simulink model "drone"  (R2018a)
settings: Solver=ode3  StartTime=0.0  StopTime=1000  FixedStep=0.05  RelTol=1e-3  EnableMultiTasking=on
PreLoadFcn:
  | init
InitFcn:
  | init
StopFcn:
  | plots
values from neighbouring files (symbols this model uses):
  cmd_phi = 0    [init.m]
  cmd_psi = 0    [init.m]
  cmd_theta = 0    [init.m]
  cmd_z = 0    [init.m]
  deltaU1_max = Kf*4	*omega_hover_max^2    [init.m]
  deltaU1_min = Kf*4	*omega_hover_min^2    [init.m]
  deltaU2_max = Kf	*omega_hover^2    [init.m]
  deltaU3_max = Kf	*omega_hover^2    [init.m]
  deltaU4_max = Km*2	*omega_hover^2    [init.m]
  g = -9.81    [init.m]
  kd_phi = 0.5    [init.m]
  kd_psi = 0.5    [init.m]
  kd_theta = 0.5    [init.m]
  kd_z = 10    [init.m]
  Kf = 1.341e-5    (= 1.341e-05)    [init.m]
  ki_phi = 0.1    [init.m]
  ki_psi = 0.2    [init.m]
  ki_theta = 0.1    [init.m]
  ki_z = 1    [init.m]
  Km = 1.465e-6    (= 1.465e-06)    [init.m]
  kp_phi = 1    [init.m]
  kp_psi = 1    [init.m]
  kp_theta = 1    [init.m]
  kp_z = 8    [init.m]
  L = 0.235    [init.m]
  m = 1.3    [init.m]
  omega_hover_max = omega_hover + omega_hover*0.20    [init.m]
  omega_hover_min = omega_hover - omega_hover*0.10    [init.m]
undefined symbols (not defined in the file or in its folder): a, b, DiscIntNeverNeededParam
libraries: simulink x1
settings Model: Creator=Felipe Vargas  LastModifiedBy=gbs
settings DataIOCC: LimitDataPoints=on  SaveFormat=Array
settings OptimizationCC: BlockReduction=off  BufferReuse=off  LifeSpan=inf
settings DebuggingCC: AlgebraicLoopMsg=none  UnconnectedInputMsg=none  UnconnectedOutputMsg=none  UnconnectedLineMsg=none  SFUnexpectedBacktrackingDiag=warning  SFNoUnconditionalDefaultTransitionDiag=warning  SFExecutionAtInitializationDiag=none
settings HardwareCC: ProdBitPerPointer=32  ProdBitPerSizeT=32  ProdBitPerPtrDiffT=32  ProdLargestAtomicFloat=None  ProdIntDivRoundTo=Undefined  ProdEndianess=Unspecified  ProdWordSize=32  ProdHWDeviceType=32-bit Generic
settings ModelReferenceCC: PropagateSignalLabelsOutOfModel=off
settings CodeAppCC: StateflowObjectComments=on
settings GRTTargetCC: TargetLangStandard=C89/C90 (ANSI)  GeneratePreprocessorConditionals=Disable all
settings ConfigComp: CovMetricSettings=dw  CovHtmlReporting=on  CovSaveCumulativeToWorkspaceVar=on  CovSaveSingleToWorkspaceVar=on  CovExternalEMLEnable=off

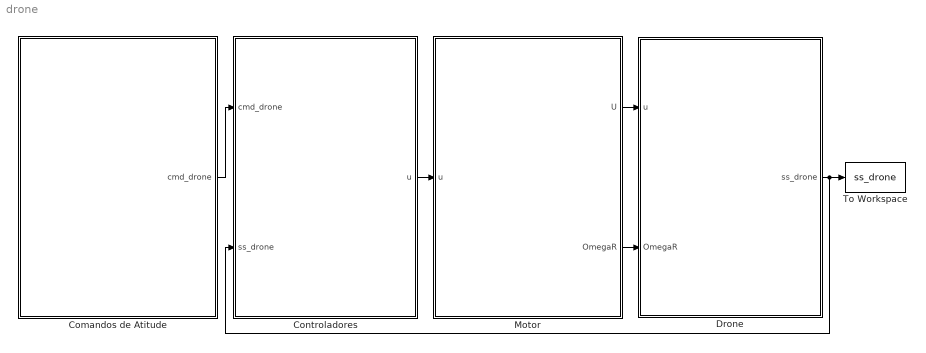
== system drone ==
  Comandos de Atitude : Subsystem
  Controladores : Subsystem
  Drone : Subsystem
  Motor : Subsystem
  To Workspace : ToWorkspace  VariableName=ss_drone  SaveFormat=Timeseries  SampleTime=-1
  wires:
  Drone/1(ss_drone) -> Controladores/2(ss_drone), To Workspace/1
  Comandos de Atitude/1(cmd_drone) -> Controladores/1(cmd_drone)
  Controladores/1(u) -> Motor/1(u)
  Motor/1(U) -> Drone/1(u)
  Motor/2(OmegaR) -> Drone/2(OmegaR)

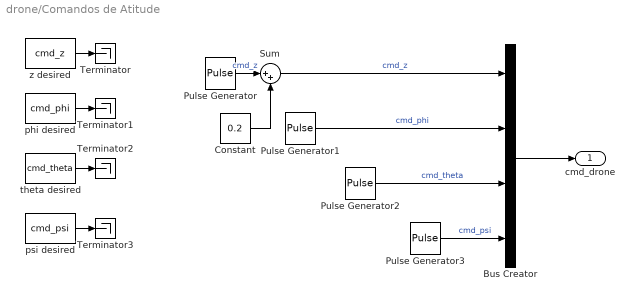
== system drone/Comandos de Atitude ==
  Bus Creator : BusCreator  Inputs=4
  Constant : Constant  Value=0.2
  Pulse Generator : DiscretePulseGenerator  PulseType=Time based  Amplitude=0.3  Period=1000  PulseWidth=10  PhaseDelay=500  SampleTime=0.05
  Pulse Generator1 : DiscretePulseGenerator  PulseType=Time based  Amplitude=0.2  Period=1000  PulseWidth=10  PhaseDelay=250  SampleTime=0.05
  Pulse Generator2 : DiscretePulseGenerator  PulseType=Time based  Amplitude=0.1  Period=1000  PulseWidth=10  PhaseDelay=50  SampleTime=0.05
  Pulse Generator3 : DiscretePulseGenerator  PulseType=Time based  Amplitude=0.1  Period=1000  PulseWidth=10  PhaseDelay=700  SampleTime=0.05
  Sum : Sum  Inputs=|++
  Terminator{,1..3} (4 alike) : Terminator
  phi desired : Constant  Value=cmd_phi
  "psi desired " : Constant  Value=cmd_psi
  theta desired : Constant  Value=cmd_theta
  z desired : Constant  Value=cmd_z
  cmd_drone : Outport
  wires:
  Bus Creator/1 -> cmd_drone/1
  Sum/1 -> Bus Creator/1  "cmd_z"
  Pulse Generator1/1 -> Bus Creator/2  "cmd_phi"
  Pulse Generator3/1 -> Bus Creator/4  "cmd_psi"
  Pulse Generator2/1 -> Bus Creator/3  "cmd_theta"
  Pulse Generator/1 -> Sum/1  "cmd_z"
  Constant/1 -> Sum/2
  z desired/1 -> Terminator/1
  phi desired/1 -> Terminator1/1
  theta desired/1 -> Terminator2/1
  "psi desired "/1 -> Terminator3/1

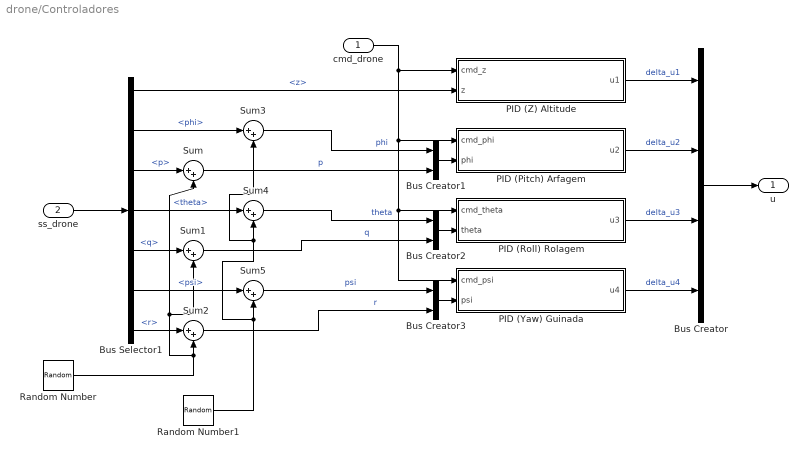
== system drone/Controladores ==
  cmd_drone : Inport
  ss_drone : Inport  Port=2
  Bus Creator : BusCreator  Inputs=4
  Bus Creator1 : BusCreator  Inputs=2
  Bus Creator2 : BusCreator  Inputs=2
  Bus Creator3 : BusCreator  Inputs=2
  Bus Selector1 : BusSelector  OutputSignals=z,phi,p,theta,q,psi,r
  PID (Pitch) Arfagem : Subsystem
  PID (Roll) Rolagem : Subsystem
  PID (Yaw) Guinada : Subsystem
  PID (Z) Altitude : Subsystem
  Random Number : RandomNumber  Variance=0.0001  SampleTime=0.05
  Random Number1 : RandomNumber  Variance=0.0001  SampleTime=0.05
  Sum{,1..5} (6 alike) : Sum  Inputs=|++
  u : Outport
  wires:
  cmd_drone/1 -> PID (Z) Altitude/1(cmd_z), PID (Pitch) Arfagem/1(cmd_phi), PID (Yaw) Guinada/1(cmd_psi), PID (Roll) Rolagem/1(cmd_theta)
  Bus Selector1/1 -> PID (Z) Altitude/2(z)  "<z>"
  PID (Z) Altitude/1(u1) -> Bus Creator/1  "delta_u1"
  PID (Pitch) Arfagem/1(u2) -> Bus Creator/2  "delta_u2"
  PID (Roll) Rolagem/1(u3) -> Bus Creator/3  "delta_u3"
  PID (Yaw) Guinada/1(u4) -> Bus Creator/4  "delta_u4"
  Bus Creator1/1 -> PID (Pitch) Arfagem/2(phi)
  Bus Creator2/1 -> PID (Roll) Rolagem/2(theta)
  Bus Creator3/1 -> PID (Yaw) Guinada/2(psi)
  Bus Selector1/2 -> Sum3/1  "<phi>"
  Bus Selector1/4 -> Sum4/1  "<theta>"
  Bus Selector1/6 -> Sum5/1  "<psi>"
  Bus Selector1/7 -> Sum2/1  "<r>"
  Bus Selector1/5 -> Sum1/1  "<q>"
  Bus Creator/1 -> u/1
  ss_drone/1 -> Bus Selector1/1
  Bus Selector1/3 -> Sum/1  "<p>"
  Sum/1 -> Bus Creator1/2  "p"
  Sum1/1 -> Bus Creator2/2  "q"
  Sum2/1 -> Bus Creator3/2  "r"
  Random Number/1 -> Sum1/2, Sum/2, Sum2/2
  Random Number1/1 -> Sum3/2, Sum4/2, Sum5/2
  Sum3/1 -> Bus Creator1/1  "phi"
  Sum4/1 -> Bus Creator2/1  "theta"
  Sum5/1 -> Bus Creator3/1  "psi"

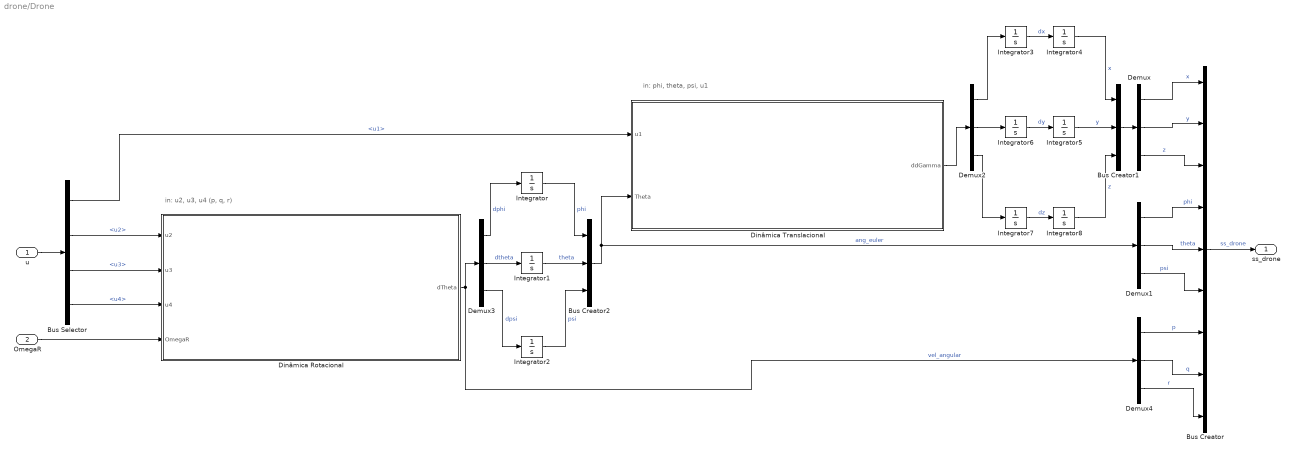
== system drone/Drone ==
  note: in: u2, u3, u4 (p, q, r)
  note: in: phi, theta, psi, u1
  u : Inport
  OmegaR : Inport  Port=2
  Bus Creator : BusCreator  Inputs=9
  Bus Creator1 : BusCreator  Inputs=3
  Bus Creator2 : BusCreator  Inputs=3
  Bus Selector : BusSelector  OutputSignals=u1,u2,u3,u4
  Demux{,1..4} (5 alike) : Demux  Outputs=3
  "Dinâmica Rotacional " : Subsystem
      mask Display: image(imread('img/u_W2euler.png'))
  Dinâmica Translacional : Subsystem
      mask Display: image(imread('img/u_euler2pos.png'))
  Integrator{,1..8} (9 alike) : Integrator
  ss_drone : Outport
  wires:
  Bus Creator/1 -> ss_drone/1  "ss_drone"
  OmegaR/1 -> "Dinâmica Rotacional "/4(OmegaR)
  Demux/1 -> Bus Creator/1  "x"
  Demux/2 -> Bus Creator/2  "y"
  Demux/3 -> Bus Creator/3  "z"
  Demux1/1 -> Bus Creator/4  "phi"
  Demux1/2 -> Bus Creator/5  "theta"
  Demux1/3 -> Bus Creator/6  "psi"
  Demux2/1 -> Integrator3/1
  Integrator3/1 -> Integrator4/1  "dx"
  Integrator4/1 -> Bus Creator1/1  "x"
  Demux2/2 -> Integrator6/1
  Integrator6/1 -> Integrator5/1  "dy"
  Integrator5/1 -> Bus Creator1/2  "y"
  Integrator7/1 -> Integrator8/1  "dz"
  Integrator8/1 -> Bus Creator1/3  "z"
  Demux2/3 -> Integrator7/1
  Dinâmica Translacional/1(ddGamma) -> Demux2/1
  Bus Creator1/1 -> Demux/1
  Demux3/1 -> Integrator/1  "dphi"
  Demux3/2 -> Integrator1/1  "dtheta"
  Demux3/3 -> Integrator2/1  "dpsi"
  "Dinâmica Rotacional "/1(dTheta) -> Demux4/1, Demux3/1  "vel_angular"
  Integrator/1 -> Bus Creator2/1  "phi"
  Integrator1/1 -> Bus Creator2/2  "theta"
  Integrator2/1 -> Bus Creator2/3  "psi"
  Demux4/1 -> Bus Creator/7  "p"
  Demux4/2 -> Bus Creator/8  "q"
  Demux4/3 -> Bus Creator/9  "r"
  Bus Creator2/1 -> Dinâmica Translacional/2(Theta), Demux1/1  "ang_euler"
  u/1 -> Bus Selector/1
  Bus Selector/1 -> Dinâmica Translacional/1(u1)  "<u1>"
  Bus Selector/2 -> "Dinâmica Rotacional "/1(u2)  "<u2>"
  Bus Selector/3 -> "Dinâmica Rotacional "/2(u3)  "<u3>"
  Bus Selector/4 -> "Dinâmica Rotacional "/3(u4)  "<u4>"

== system drone/Motor ==
  note: Omega ---> Omega_real
  note: U ---> Omega^2 ---> Omega
  u : Inport
  Cálculos das Velocidades de Rotação : Subsystem
      mask Display: image(imread('img/u2w.png'))
  Cálculos dos Comandos Reais : Subsystem
      mask Display: image(imread('img/om_actual2u.PNG'))
  Motor Dynamics : Subsystem
  To Workspace : ToWorkspace  VariableName=w  SaveFormat=Timeseries  SampleTime=-1
  U : Outport
  OmegaR : Outport  Port=2
  wires:
  u/1 -> Cálculos das Velocidades de Rotação/1(u)
  Cálculos das Velocidades de Rotação/2(OmegaR) -> OmegaR/1
  Cálculos das Velocidades de Rotação/1(omega) -> Motor Dynamics/1(om_desired)
  Motor Dynamics/1(om_actual) -> To Workspace/1, Cálculos dos Comandos Reais/1(om_Actual)
  Cálculos dos Comandos Reais/1(u_actual) -> U/1

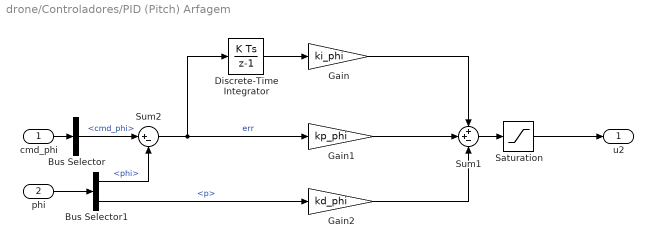
== system drone/Controladores/PID (Pitch) Arfagem ==
  cmd_phi : Inport
  phi : Inport  Port=2
  Bus Selector : BusSelector  OutputSignals=cmd_phi
  Bus Selector1 : BusSelector  OutputSignals=phi,p
  Discrete-Time Integrator : DiscreteIntegrator  SampleTime=0.05  LimitOutput=on  UpperSaturationLimit=1  LowerSaturationLimit=-1  ICPrevOutput=DiscIntNeverNeededParam  ICPrevScaledInput=DiscIntNeverNeededParam
  Gain : Gain  Gain=ki_phi
  Gain1 : Gain  Gain=kp_phi
  Gain2 : Gain  Gain=kd_phi
  Saturation : Saturate  UpperLimit=deltaU2_max  LowerLimit=-deltaU3_max
  Sum1 : Sum  Inputs=++-
  Sum2 : Sum  Inputs=|+-
  u2 : Outport
  wires:
  Sum2/1 -> Discrete-Time Integrator/1, Gain1/1  "err"
  Sum1/1 -> Saturation/1
  Gain/1 -> Sum1/1
  Gain2/1 -> Sum1/3
  Gain1/1 -> Sum1/2
  Saturation/1 -> u2/1
  Discrete-Time Integrator/1 -> Gain/1
  cmd_phi/1 -> Bus Selector/1
  Bus Selector/1 -> Sum2/1  "<cmd_phi>"
  phi/1 -> Bus Selector1/1
  Bus Selector1/1 -> Sum2/2  "<phi>"
  Bus Selector1/2 -> Gain2/1  "<p>"

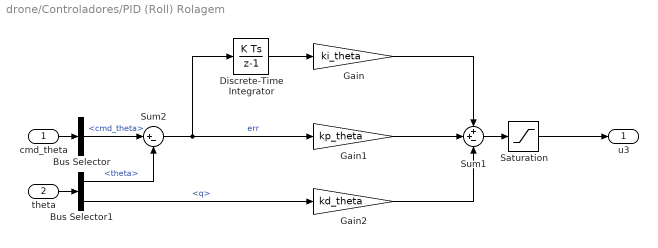
== system drone/Controladores/PID (Roll) Rolagem ==
  cmd_theta : Inport
  theta : Inport  Port=2
  Bus Selector : BusSelector  OutputSignals=cmd_theta
  Bus Selector1 : BusSelector  OutputSignals=theta,q
  Discrete-Time Integrator : DiscreteIntegrator  SampleTime=0.05  LimitOutput=on  UpperSaturationLimit=1  LowerSaturationLimit=-1  ICPrevOutput=DiscIntNeverNeededParam  ICPrevScaledInput=DiscIntNeverNeededParam
  Gain : Gain  Gain=ki_theta
  Gain1 : Gain  Gain=kp_theta
  Gain2 : Gain  Gain=kd_theta
  Saturation : Saturate  UpperLimit=deltaU3_max  LowerLimit=-deltaU3_max
  Sum1 : Sum  Inputs=++-
  Sum2 : Sum  Inputs=|+-
  u3 : Outport
  wires:
  Sum2/1 -> Discrete-Time Integrator/1, Gain1/1  "err"
  Sum1/1 -> Saturation/1
  Gain/1 -> Sum1/1
  Gain2/1 -> Sum1/3
  Gain1/1 -> Sum1/2
  Saturation/1 -> u3/1
  Discrete-Time Integrator/1 -> Gain/1
  cmd_theta/1 -> Bus Selector/1
  Bus Selector/1 -> Sum2/1  "<cmd_theta>"
  theta/1 -> Bus Selector1/1
  Bus Selector1/1 -> Sum2/2  "<theta>"
  Bus Selector1/2 -> Gain2/1  "<q>"

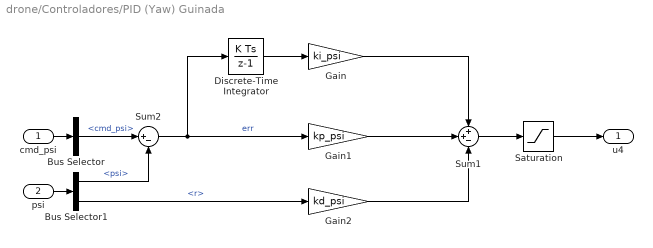
== system drone/Controladores/PID (Yaw) Guinada ==
  cmd_psi : Inport
  psi : Inport  Port=2
  Bus Selector : BusSelector  OutputSignals=cmd_psi
  Bus Selector1 : BusSelector  OutputSignals=psi,r
  Discrete-Time Integrator : DiscreteIntegrator  SampleTime=0.05  LimitOutput=on  UpperSaturationLimit=1  LowerSaturationLimit=-1  ICPrevOutput=DiscIntNeverNeededParam  ICPrevScaledInput=DiscIntNeverNeededParam
  Gain : Gain  Gain=ki_psi
  Gain1 : Gain  Gain=kp_psi
  Gain2 : Gain  Gain=kd_psi
  Saturation : Saturate  UpperLimit=deltaU4_max  LowerLimit=-deltaU4_max
  Sum1 : Sum  Inputs=++-
  Sum2 : Sum  Inputs=|+-
  u4 : Outport
  wires:
  Sum2/1 -> Discrete-Time Integrator/1, Gain1/1  "err"
  Sum1/1 -> Saturation/1
  Gain/1 -> Sum1/1
  Gain2/1 -> Sum1/3
  Gain1/1 -> Sum1/2
  Saturation/1 -> u4/1
  Discrete-Time Integrator/1 -> Gain/1
  cmd_psi/1 -> Bus Selector/1
  Bus Selector/1 -> Sum2/1  "<cmd_psi>"
  psi/1 -> Bus Selector1/1
  Bus Selector1/1 -> Sum2/2  "<psi>"
  Bus Selector1/2 -> Gain2/1  "<r>"

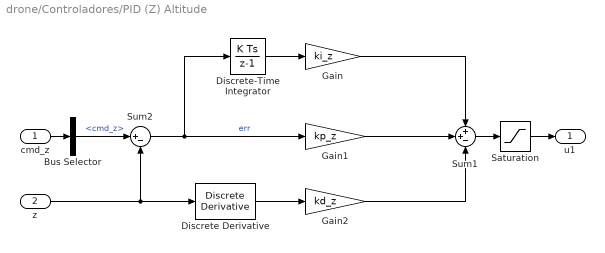
== system drone/Controladores/PID (Z) Altitude ==
  cmd_z : Inport
  z : Inport  Port=2
  Bus Selector : BusSelector  OutputSignals=cmd_z
  Discrete Derivative : simulink/Discrete/Discrete Derivative  gainval=1.0  ICPrevScaledInput=0.0  InputProcessing=Inherited  OutMin=[]  OutMax=[]  OutDataType=fixdt(1, 16)  OutScaling=2^-10  DoSatur=off
  Discrete-Time Integrator : DiscreteIntegrator  SampleTime=0.05  LimitOutput=on  UpperSaturationLimit=20  LowerSaturationLimit=-20  ICPrevOutput=DiscIntNeverNeededParam  ICPrevScaledInput=DiscIntNeverNeededParam
  Gain : Gain  Gain=ki_z
  Gain1 : Gain  Gain=kp_z
  Gain2 : Gain  Gain=kd_z
  Saturation : Saturate  UpperLimit=deltaU1_max  LowerLimit=deltaU1_min
  Sum1 : Sum  Inputs=++-
  Sum2 : Sum  Inputs=|+-
  u1 : Outport
  wires:
  z/1 -> Discrete Derivative/1, Sum2/2
  Sum2/1 -> Discrete-Time Integrator/1, Gain1/1  "err"
  Sum1/1 -> Saturation/1
  Gain2/1 -> Sum1/3
  Discrete Derivative/1 -> Gain2/1
  Gain1/1 -> Sum1/2
  Saturation/1 -> u1/1
  Discrete-Time Integrator/1 -> Gain/1
  cmd_z/1 -> Bus Selector/1
  Bus Selector/1 -> Sum2/1  "<cmd_z>"
  Gain/1 -> Sum1/1

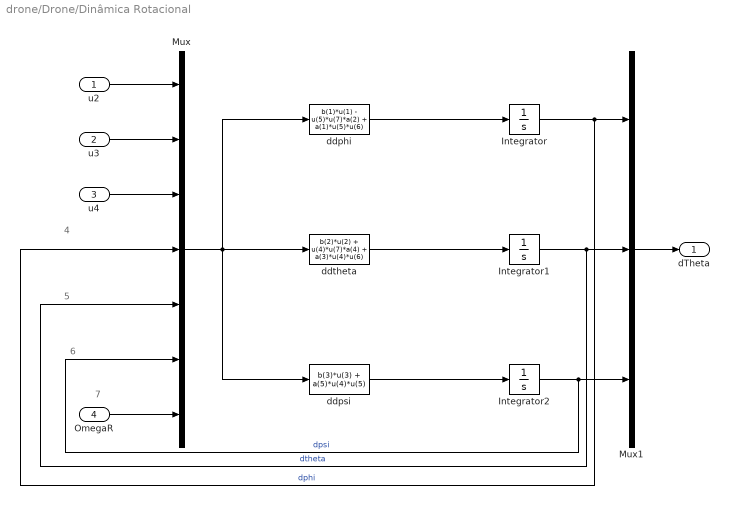
== system drone/Drone/Dinâmica Rotacional  ==
  note: 7
  note: 6
  note: 5
  note: 4
  u2 : Inport
  u3 : Inport  Port=2
  u4 : Inport  Port=3
  OmegaR : Inport  Port=4
  Integrator : Integrator
  Integrator1 : Integrator
  Integrator2 : Integrator
  Mux : Mux  Inputs=7
  Mux1 : Mux  Inputs=3
  ddphi : Fcn  Expr=b(1)*u(1) - u(5)*u(7)*a(2) + a(1)*u(5)*u(6)
  ddpsi : Fcn  Expr=b(3)*u(3) + a(5)*u(4)*u(5)
  ddtheta : Fcn  Expr=b(2)*u(2) + u(4)*u(7)*a(4) + a(3)*u(4)*u(6)
  dTheta : Outport
  wires:
  u2/1 -> Mux/1
  u3/1 -> Mux/2
  u4/1 -> Mux/3
  Integrator/1 -> Mux1/1, Mux/4  "dphi"
  Mux/1 -> ddpsi/1, ddtheta/1, ddphi/1
  Integrator1/1 -> Mux1/2, Mux/5  "dtheta"
  Integrator2/1 -> Mux1/3, Mux/6  "dpsi"
  Mux1/1 -> dTheta/1
  OmegaR/1 -> Mux/7
  ddpsi/1 -> Integrator2/1
  ddtheta/1 -> Integrator1/1
  ddphi/1 -> Integrator/1

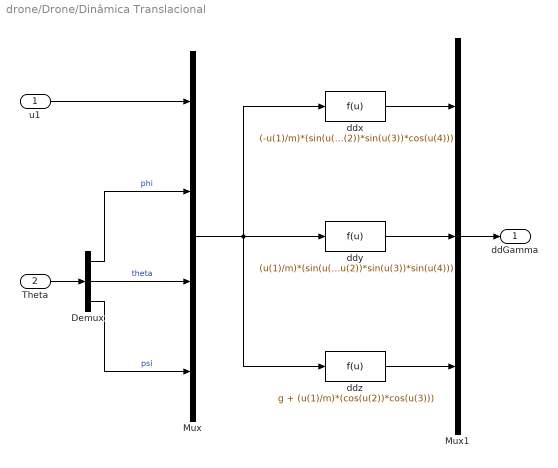
== system drone/Drone/Dinâmica Translacional ==
  u1 : Inport
  Theta : Inport  Port=2
  Demux : Demux  Outputs=3
  Mux : Mux
  Mux1 : Mux  Inputs=3
  ddx : Fcn  Expr=(-u(1)/m)*(sin(u(2))*sin(u(4)) + cos(u(2))*sin(u(3))*cos(u(4)))
  ddy : Fcn  Expr=(u(1)/m)*(sin(u(2))*cos(u(4)) - cos(u(2))*sin(u(3))*sin(u(4)))
  ddz : Fcn  Expr=g + (u(1)/m)*(cos(u(2))*cos(u(3)))
  ddGamma : Outport
  wires:
  Mux1/1 -> ddGamma/1
  Theta/1 -> Demux/1
  Mux/1 -> ddz/1, ddy/1, ddx/1
  u1/1 -> Mux/1
  Demux/1 -> Mux/2  "phi"
  Demux/2 -> Mux/3  "theta"
  Demux/3 -> Mux/4  "psi"
  ddy/1 -> Mux1/2
  ddx/1 -> Mux1/1
  ddz/1 -> Mux1/3

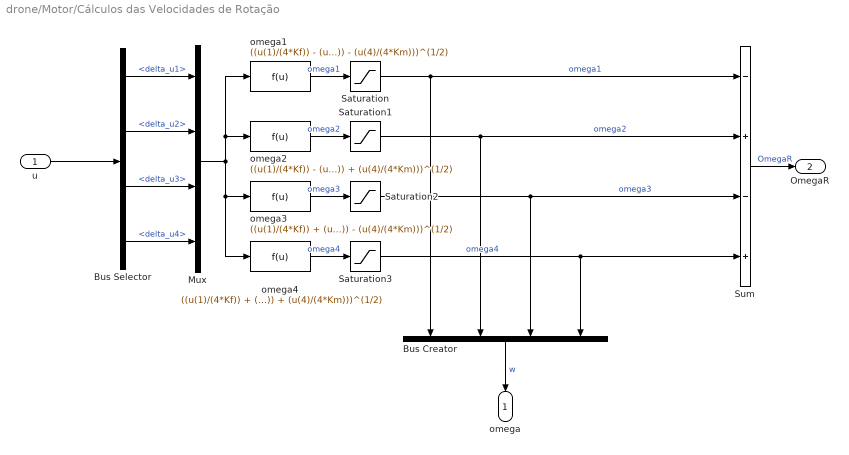
== system drone/Motor/Cálculos das Velocidades de Rotação ==
  u : Inport
  Bus Creator : BusCreator  Inputs=4
  Bus Selector : BusSelector  OutputSignals=delta_u1,delta_u2,delta_u3,delta_u4
  Mux : Mux
  Saturation{,1..3} (4 alike) : Saturate  UpperLimit=omega_hover_max  LowerLimit=omega_hover_min
  Sum : Sum  Inputs=-+-+
  omega1 : Fcn  Expr=((u(1)/(4*Kf)) - (u(3)/(2*Kf*L)) - (u(4)/(4*Km)))^(1/2)
  omega2 : Fcn  Expr=((u(1)/(4*Kf)) - (u(2)/(2*Kf*L)) + (u(4)/(4*Km)))^(1/2)
  omega3 : Fcn  Expr=((u(1)/(4*Kf)) + (u(3)/(2*Kf*L)) - (u(4)/(4*Km)))^(1/2)
  omega4 : Fcn  Expr=((u(1)/(4*Kf)) + (u(2)/(2*Kf*L)) + (u(4)/(4*Km)))^(1/2)
  omega : Outport
  OmegaR : Outport  Port=2
  wires:
  omega2/1 -> Saturation1/1  "omega2"
  omega1/1 -> Saturation/1  "omega1"
  omega3/1 -> Saturation2/1  "omega3"
  Mux/1 -> omega1/1, omega2/1, omega4/1, omega3/1
  omega4/1 -> Saturation3/1  "omega4"
  Sum/1 -> OmegaR/1  "OmegaR"
  Bus Creator/1 -> omega/1  "w"
  u/1 -> Bus Selector/1
  Bus Selector/1 -> Mux/1  "<delta_u1>"
  Bus Selector/2 -> Mux/2  "<delta_u2>"
  Bus Selector/3 -> Mux/3  "<delta_u3>"
  Bus Selector/4 -> Mux/4  "<delta_u4>"
  Saturation/1 -> Bus Creator/1, Sum/1  "omega1"
  Saturation1/1 -> Bus Creator/2, Sum/2  "omega2"
  Saturation2/1 -> Bus Creator/3, Sum/3  "omega3"
  Saturation3/1 -> Bus Creator/4, Sum/4  "omega4"

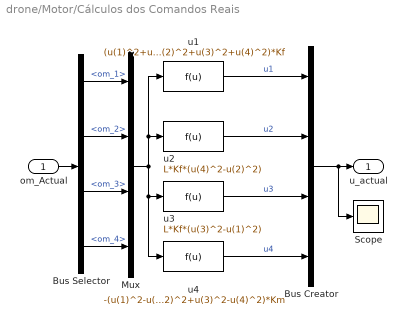
== system drone/Motor/Cálculos dos Comandos Reais ==
  om_Actual : Inport
  Bus Creator : BusCreator  Inputs=4
  Bus Selector : BusSelector  OutputSignals=om_1,om_2,om_3,om_4
  Mux : Mux
  Scope : Scope
  u1 : Fcn  Expr=(u(1)^2+u(2)^2+u(3)^2+u(4)^2)*Kf
  u2 : Fcn  Expr=L*Kf*(u(4)^2-u(2)^2)
  u3 : Fcn  Expr=L*Kf*(u(3)^2-u(1)^2)
  u4 : Fcn  Expr=-(u(1)^2-u(2)^2+u(3)^2-u(4)^2)*Km
  u_actual : Outport
  wires:
  Bus Selector/4 -> Mux/4  "<om_4>"
  Bus Selector/3 -> Mux/3  "<om_3>"
  Bus Selector/2 -> Mux/2  "<om_2>"
  Bus Selector/1 -> Mux/1  "<om_1>"
  om_Actual/1 -> Bus Selector/1
  Bus Creator/1 -> Scope/1, u_actual/1
  u4/1 -> Bus Creator/4  "u4"
  u1/1 -> Bus Creator/1  "u1"
  u3/1 -> Bus Creator/3  "u3"
  u2/1 -> Bus Creator/2  "u2"
  Mux/1 -> u4/1, u3/1, u1/1, u2/1

== system drone/Motor/Motor Dynamics ==
  om_desired : Inport
  Bus Creator : BusCreator  Inputs=4
  Bus Selector : BusSelector  OutputSignals=omega1,omega2,omega3,omega4
  Transfer Fcn{,1..3} (4 alike) : TransferFcn  Numerator=[0.936]  Denominator=[0.178 1]
  om_actual : Outport
  wires:
  Transfer Fcn3/1 -> Bus Creator/4  "om_4"
  Transfer Fcn2/1 -> Bus Creator/3  "om_3"
  Transfer Fcn1/1 -> Bus Creator/2  "om_2"
  Bus Selector/2 -> Transfer Fcn1/1  "<omega2>"
  Bus Selector/3 -> Transfer Fcn2/1  "<omega3>"
  Bus Selector/4 -> Transfer Fcn3/1  "<omega4>"
  Transfer Fcn/1 -> Bus Creator/1  "om_1"
  Bus Selector/1 -> Transfer Fcn/1  "<omega1>"
  om_desired/1 -> Bus Selector/1
  Bus Creator/1 -> om_actual/1
